simulink model "Simulink_Lab1"  (R2014a)
settings: Solver=ode45  StartTime=0.0  StopTime=10.0  RelTol=1e-3
settings Model: Creator=Omar Emad  LastModifiedBy=Omar Emad

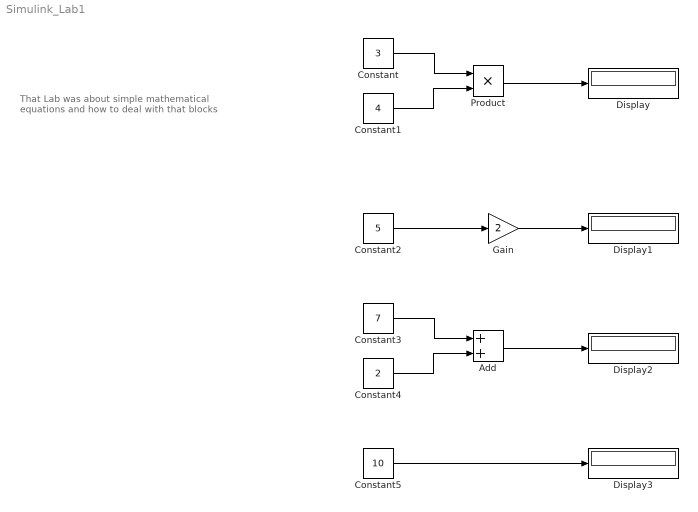
== system Simulink_Lab1 ==
  note: That Lab was about simple mathematical
      | equations and how to deal with that blocks
  Add : Sum
  Constant : Constant  Value=3
  Constant1 : Constant  Value=4
  Constant2 : Constant  Value=5
  Constant3 : Constant  Value=7
  Constant4 : Constant  Value=2
  Constant5 : Constant  Value=10
  Display{,1..3} (4 alike) : Display
  Gain : Gain  Gain=2
  Product : Product
  wires:
  Product/1 -> Display/1
  Constant/1 -> Product/1
  Constant1/1 -> Product/2
  Constant2/1 -> Gain/1
  Gain/1 -> Display1/1
  Add/1 -> Display2/1
  Constant3/1 -> Add/1
  Constant4/1 -> Add/2
  Constant5/1 -> Display3/1
